simulink model "gm_sampleModel1444_3_sub"  (R2023a)
settings: Solver=VariableStepAuto  StartTime=0.0  StopTime=10.0  RelTol=1e-3
libraries: simulink x2, hdlsllib x1
settings Model: Creator=user1  LastModifiedBy=user1
settings OptimizationCC: BlockReduction=off  ConditionallyExecuteInputs=off
settings DebuggingCC: InheritedTsInSrcMsg=none

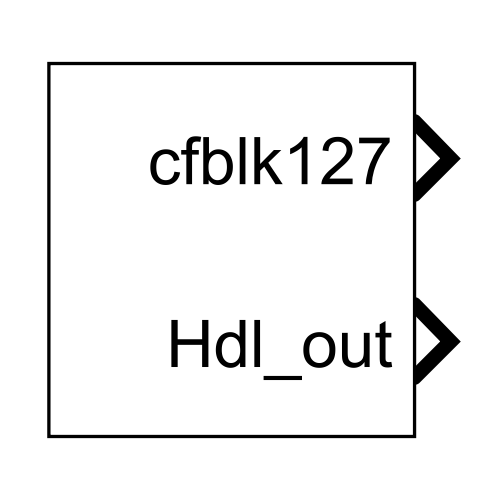
[thumbnail: Simulink's stored preview of the top-level diagram]
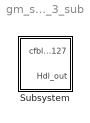
== system gm_sampleModel1444_3_sub ==
  Subsystem : Subsystem

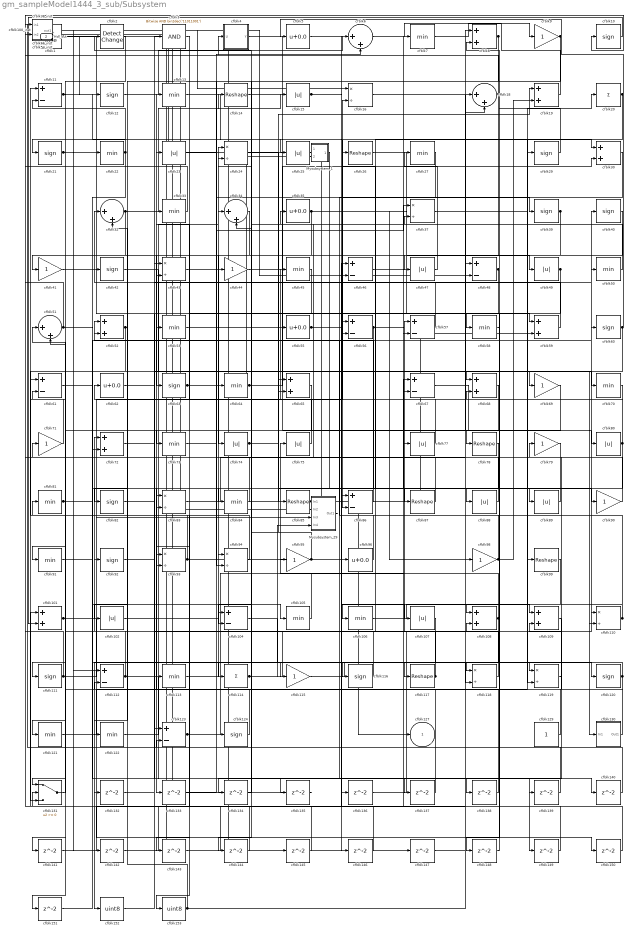
== system gm_sampleModel1444_3_sub/Subsystem ==
  Mysubsystem_1 : Subsystem
  Mysubsystem_29 : Subsystem
  cfblk1 : hdlsllib/Logic and Bit Operations/Bit Slice  lidx=7  ridx=0
  cfblk{10,12,21,29,39..40,42,60,63,82,92,111,116,120,124} (15 alike) : Signum
  cfblk100_inst : Subsystem
  cfblk{8,19,30,52,59,65,68,72,101,108..109} (11 alike) : Sum  OutDataTypeStr=uint8
  cfblk{15,23,25,47,49,74..75,77,80,88..89,102,107} (13 alike) : Abs  OutDataTypeStr=uint8  SaturateOnIntegerOverflow=off
  cfblk{11,46,48,56..57,61,67,86,104,112,123} (11 alike) : Sum  Inputs=+-  OutDataTypeStr=uint8
  cfblk{7,13,22,27,33,45,50,53,58,64,70,73,81,84,91,105..106,113,121..122} (20 alike) : MinMax  OutDataTypeStr=uint8
  cfblk{16,24,37,43,83,93..94,110,118..119} (10 alike) : Product  Inputs=*/  OutDataTypeStr=uint8  RndMeth=Zero  SaturateOnIntegerOverflow=on
  cfblk114 : Sum  Inputs=+  OutDataTypeStr=uint8
  cfblk{9,41,44,69,71,79,90,95,98,115} (10 alike) : Gain  OutDataTypeStr=uint8
  cfblk{14,26,78,85,87,99,117} (7 alike) : Reshape
  cfblk129 : Constant  OutDataTypeStr=uint8  SampleTime=-1
  cfblk130 : Subsystem
  cfblk131 : Switch  OutDataTypeStr=uint8  SaturateOnIntegerOverflow=off  InputSameDT=off
  cfblk{132..151} (20 alike) : Delay  SampleTime=1
  cfblk152 : DataTypeConversion  OutDataTypeStr=uint8  SaturateOnIntegerOverflow=off  RndMeth=Floor
  cfblk153 : DataTypeConversion  OutDataTypeStr=uint8  SaturateOnIntegerOverflow=off  RndMeth=Floor
  cfblk{6,18,32,34,51} (5 alike) : Sum  Inputs=|++  OutDataTypeStr=uint8
  cfblk2 : simulink/Logic and Bit Operations/Detect Change  vinit=0  OutDataTypeStr=uint8
      settings: LibrarySourceBlock=|
      | hdlsllib/Logic and Bit
      | Operations/Detect
      | Change
  cfblk20 : Sum  Inputs=+  OutDataTypeStr=uint8
  cfblk3 : simulink/Logic and Bit Operations/Bitwise Operator  logicop=AND  UseBitMask=on  BitMask=bin2dec('11011001')  BitMaskRealWorld=Stored Integer
      settings: LibrarySourceBlock=|
      | hdlsllib/Logic and Bit
      | Operations/Bitwise
      | Operator
  cfblk{5,35,55,62,96} (5 alike) : Bias  Bias=0.0  SaturateOnIntegerOverflow=off
  cfblk38_inst : Subsystem
  cfblk4 : Subsystem  mask(Detect Rise Nonnegative){vinit=double(0), InputProcessing=Elements as channels (sample based), OutDataTypeStr=uint8}
      mask prompts: vinit "Simulink:masks:InitialCondition_MP"; InputProcessing "Simulink:masks:InputProcessing_MP"; OutDataTypeStr "Simulink:masks:OutputDataType_MP"
      mask help: Simulink:masks:DetectRiseNonnegative_MD
      mask init:
      | InputProcessing = 'Elements as channels (sample based)';
      | OutDataTypeStr = 'uint8';
      | vinit = double(0);
      mask TypeOptions InputProcessing: Simulink:masks:ColumnsAsChannelsFrameBased | Simulink:masks:ElementsAsChannelsSampleBased
      mask TypeOptions OutDataTypeStr: Simulink:masks:uint8 | Simulink:masks:boolean
      mask Display: fprintf('U >= 0\n&  NOT\nU/z >= 0')
  cfblk54_inst : Subsystem
  cfblk66_inst : Subsystem
  cfblk127 : Outport  OutDataTypeStr=uint8  SampleTime=1  VectorParamsAs1DForOutWhenUnconnected=off
  Hdl_out : Outport  Port=2  OutDataTypeStr=uint8  SampleTime=1
  wires:
  Mysubsystem_1/1(Out1) -> cfblk133/1
  Mysubsystem_29/1(Out1) -> Mysubsystem_1/1(In1)
  cfblk1/1 -> cfblk86/2, cfblk12/1
  cfblk10/1 -> cfblk101/2
  cfblk100_inst/1(out1) -> cfblk48/2, Mysubsystem_29/2(In2)
  cfblk101/1 -> cfblk150/1, Mysubsystem_29/3(In3), cfblk105/1
  cfblk102/1 -> cfblk24/1
  cfblk104/1 -> cfblk119/1
  cfblk105/1 -> cfblk75/1
  cfblk106/1 -> cfblk109/1
  cfblk107/1 -> cfblk152/1
  cfblk108/1 -> cfblk95/1, cfblk132/1
  cfblk109/1 -> cfblk134/1
  cfblk11/1 -> cfblk30/1, cfblk151/1
  cfblk110/1 -> cfblk62/1, cfblk108/1
  cfblk111/1 -> cfblk10/1, cfblk16/2
  cfblk112/1 -> cfblk72/1, cfblk149/1
  cfblk113/1 -> cfblk94/1
  cfblk114/1 -> cfblk40/1, Mysubsystem_29/4(In4)
  cfblk115/1 -> cfblk120/1
  cfblk116/1 -> cfblk61/2
  cfblk117/1 -> cfblk92/1, cfblk57/1
  cfblk118/1 -> cfblk26/1
  cfblk119/1 -> cfblk79/1
  cfblk12/1 -> cfblk6/1
  cfblk120/1 -> cfblk116/1, cfblk112/2
  cfblk121/1 -> cfblk29/1
  cfblk122/1 -> cfblk34/1
  cfblk123/1 -> cfblk77/1, cfblk124/1
  cfblk124/1 -> cfblk13/1
  cfblk129/1 -> cfblk52/1
  cfblk13/1 -> cfblk96/1
  cfblk130/1(Out1) -> cfblk109/2
  cfblk131/1 -> cfblk81/1
  cfblk132/1 -> cfblk110/1
  cfblk133/1 -> cfblk6/2
  cfblk134/1 -> cfblk34/2
  cfblk135/1 -> cfblk1/1
  cfblk136/1 -> cfblk108/2
  cfblk137/1 -> cfblk93/2
  cfblk138/1 -> cfblk51/1
  cfblk139/1 -> cfblk100_inst/1(in1)
  cfblk14/1 -> cfblk146/1
  cfblk140/1 -> cfblk24/2
  cfblk141/1 -> cfblk67/1
  cfblk142/1 -> cfblk48/1
  cfblk143/1 -> cfblk46/1
  cfblk144/1 -> cfblk123/2
  cfblk145/1 -> cfblk66_inst/1(in1)
  cfblk146/1 -> cfblk101/1
  cfblk147/1 -> cfblk18/1
  cfblk148/1 -> cfblk8/2
  cfblk149/1 -> cfblk83/2
  cfblk15/1 -> cfblk59/1, cfblk69/1
  cfblk150/1 -> cfblk131/2
  cfblk151/1 -> cfblk56/2
  cfblk152/1 -> cfblk3/1
  cfblk153/1 -> cfblk52/2, cfblk18/2
  cfblk16/1 -> cfblk80/1
  cfblk18/1 -> cfblk131/1, cfblk4/1(U)
  cfblk19/1 -> cfblk7/1
  cfblk2/1 -> cfblk141/1
  cfblk20/1 -> cfblk86/1, cfblk119/2
  cfblk21/1 -> cfblk25/1, cfblk123/1
  cfblk22/1 -> cfblk72/2, cfblk21/1, cfblk11/2
  cfblk23/1 -> cfblk39/1
  cfblk24/1 -> cfblk56/1
  cfblk25/1 -> cfblk38_inst/2(in2)
  cfblk26/1 -> cfblk58/1
  cfblk27/1 -> cfblk46/2
  cfblk29/1 -> cfblk54_inst/1(in1)
  cfblk3/1 -> cfblk153/1
  cfblk30/1 -> cfblk115/1
  cfblk32/1 -> cfblk14/1, cfblk41/1
  cfblk33/1 -> cfblk100_inst/2(in2)
  cfblk34/1 -> cfblk63/1
  cfblk35/1 -> cfblk82/1, cfblk49/1, cfblk98/1
  cfblk37/1 -> cfblk20/1
  cfblk38_inst/1(out1) -> cfblk16/1, cfblk145/1, cfblk142/1
  cfblk39/1 -> cfblk47/1, cfblk37/2
  cfblk4/1(Y) -> cfblk99/1
  cfblk40/1 -> cfblk74/1
  cfblk41/1 -> cfblk85/1
  cfblk42/1 -> cfblk130/1(In1)
  cfblk43/1 -> cfblk64/1
  cfblk44/1 -> cfblk68/1
  cfblk45/1 -> cfblk143/1
  cfblk46/1 -> cfblk89/1
  cfblk47/1 -> cfblk27/1
  cfblk48/1 -> cfblk57/2, cfblk73/1
  cfblk49/1 -> cfblk104/2, cfblk148/1
  cfblk5/1 -> cfblk107/1
  cfblk50/1 -> cfblk2/1
  cfblk51/1 -> cfblk66_inst/2(in2), cfblk137/1
  cfblk52/1 -> cfblk32/2, cfblk121/1
  cfblk53/1 -> cfblk136/1
  cfblk54_inst/1(out1) -> cfblk147/1
  cfblk55/1 -> cfblk117/1, cfblk140/1
  cfblk56/1 -> cfblk93/1, cfblk90/1
  cfblk57/1 -> cfblk32/1
  cfblk58/1 -> cfblk138/1
  cfblk59/1 -> cfblk23/1
  cfblk6/1 -> cfblk67/2
  cfblk60/1 -> cfblk5/1, cfblk131/3
  cfblk61/1 -> cfblk53/1
  cfblk62/1 -> cfblk70/1
  cfblk63/1 -> cfblk37/1, Mysubsystem_1/2(In2)
  cfblk64/1 -> cfblk78/1, cfblk30/2
  cfblk65/1 -> cfblk91/1
  cfblk66_inst/1(out1) -> cfblk112/1, Mysubsystem_29/1(In1), cfblk22/1
  cfblk67/1 -> cfblk110/2
  cfblk68/1 -> cfblk122/1
  cfblk69/1 -> cfblk111/1
  cfblk7/1 -> cfblk9/1
  cfblk70/1 -> cfblk68/2
  cfblk71/1 -> cfblk11/1
  cfblk72/1 -> cfblk118/1
  cfblk73/1 -> cfblk15/1
  cfblk74/1 -> cfblk87/1, cfblk19/1
  cfblk75/1 -> cfblk43/2
  cfblk77/1 -> cfblk33/1
  cfblk78/1 -> cfblk114/1
  cfblk79/1 -> cfblk135/1
  cfblk8/1 -> cfblk102/1, cfblk94/2
  cfblk80/1 -> cfblk144/1, cfblk45/1
  cfblk81/1 -> cfblk104/1, cfblk83/1
  cfblk82/1 -> cfblk139/1
  cfblk83/1 -> cfblk8/1
  cfblk84/1 -> cfblk54_inst/2(in2)
  cfblk85/1 -> cfblk59/2, cfblk127/1
  cfblk86/1 -> cfblk42/1
  cfblk87/1 -> cfblk35/1
  cfblk88/1 -> cfblk38_inst/1(in1)
  cfblk89/1 -> cfblk88/1
  cfblk9/1 -> cfblk113/1, cfblk84/1
  cfblk90/1 -> cfblk43/1
  cfblk91/1 -> cfblk118/2
  cfblk92/1 -> cfblk50/1
  cfblk93/1 -> cfblk51/2, cfblk71/1
  cfblk94/1 -> cfblk61/1
  cfblk95/1 -> cfblk65/2, cfblk60/1, cfblk44/1, Hdl_out/1
  cfblk96/1 -> cfblk65/1
  cfblk98/1 -> cfblk55/1, cfblk19/2
  cfblk99/1 -> cfblk106/1

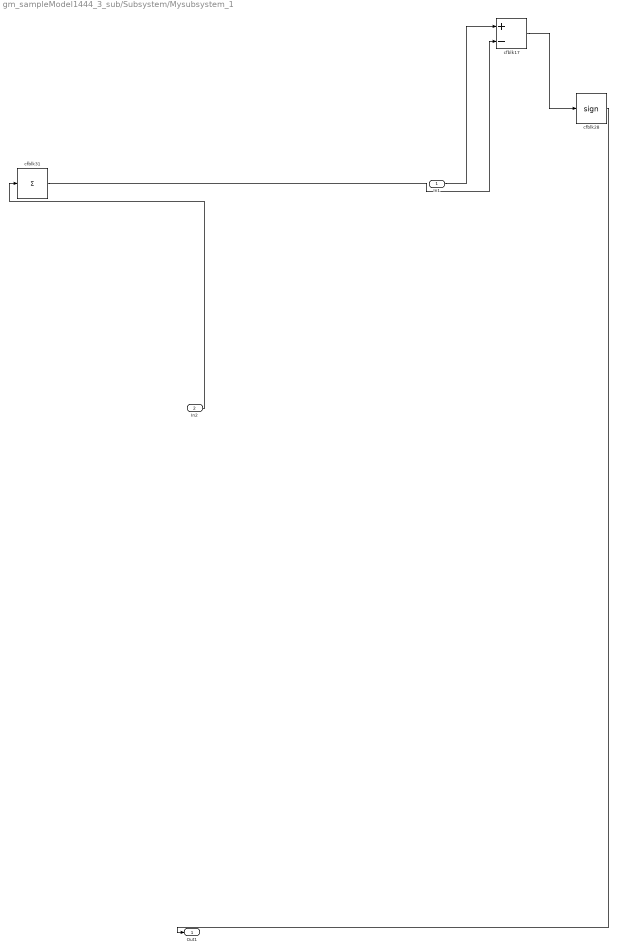
== system gm_sampleModel1444_3_sub/Subsystem/Mysubsystem_1 ==
  In1 : Inport  OutDataTypeStr=uint8  PortDimensions=1  SampleTime=1
  In2 : Inport  Port=2  OutDataTypeStr=uint8  PortDimensions=1  SampleTime=1
  cfblk17 : Sum  Inputs=+-
  cfblk28 : Signum
  cfblk31 : Sum  Inputs=+
  Out1 : Outport  SampleTime=1
  wires:
  In1/1 -> cfblk17/1
  In2/1 -> cfblk31/1
  cfblk17/1 -> cfblk28/1
  cfblk28/1 -> Out1/1
  cfblk31/1 -> cfblk17/2

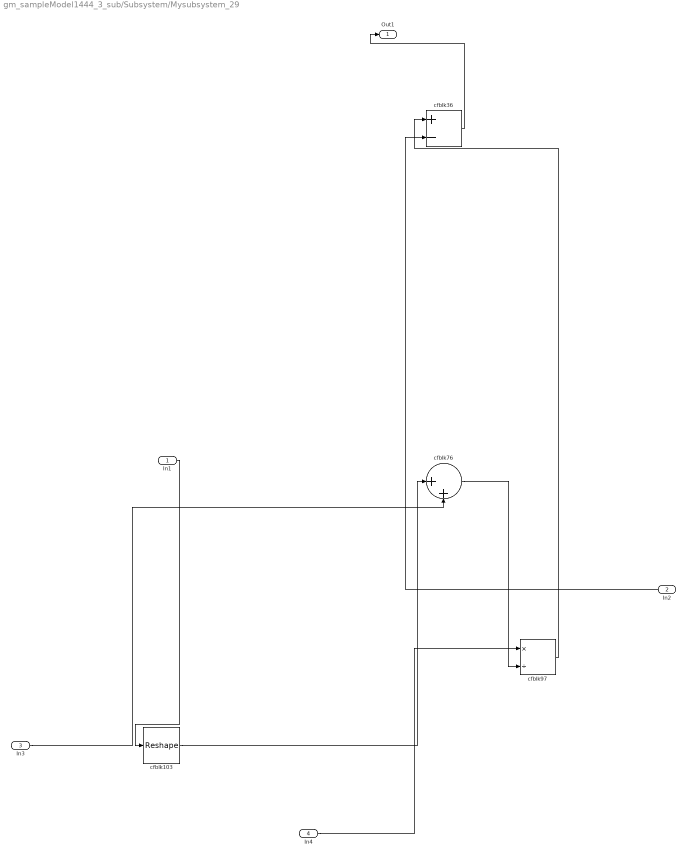
== system gm_sampleModel1444_3_sub/Subsystem/Mysubsystem_29 ==
  In1 : Inport  OutDataTypeStr=uint8  PortDimensions=1  SampleTime=1
  In2 : Inport  Port=2  OutDataTypeStr=uint8  PortDimensions=1  SampleTime=1
  In3 : Inport  Port=3  OutDataTypeStr=uint8  PortDimensions=1  SampleTime=1
  In4 : Inport  Port=4  OutDataTypeStr=uint8  PortDimensions=1  SampleTime=1
  cfblk103 : Reshape
  cfblk36 : Sum  Inputs=+-
  cfblk76 : Sum  Inputs=|++
  cfblk97 : Product  Inputs=*/  RndMeth=Zero  SaturateOnIntegerOverflow=on
  Out1 : Outport  SampleTime=1
  wires:
  In1/1 -> cfblk103/1
  In2/1 -> cfblk36/2
  In3/1 -> cfblk76/2
  In4/1 -> cfblk97/1
  cfblk103/1 -> cfblk76/1
  cfblk36/1 -> Out1/1
  cfblk76/1 -> cfblk97/2
  cfblk97/1 -> cfblk36/1

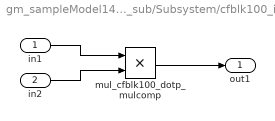
== system gm_sampleModel1444_3_sub/Subsystem/cfblk100_inst ==
  in1 : Inport  OutDataTypeStr=uint8  SampleTime=1
  in2 : Inport  Port=2  OutDataTypeStr=uint8  SampleTime=1
  mul_cfblk100_dotp_mulcomp : Product  Inputs=**  OutDataTypeStr=uint8  SampleTime=1
  out1 : Outport  OutDataTypeStr=uint8  SampleTime=1
  wires:
  in1/1 -> mul_cfblk100_dotp_mulcomp/1
  in2/1 -> mul_cfblk100_dotp_mulcomp/2
  mul_cfblk100_dotp_mulcomp/1 -> out1/1

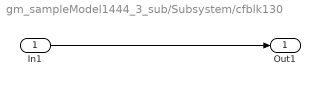
== system gm_sampleModel1444_3_sub/Subsystem/cfblk130 ==
  In1 : Inport  OutDataTypeStr=uint8  PortDimensions=1  SampleTime=1
  Out1 : Outport  SampleTime=1
  wires:
  In1/1 -> Out1/1

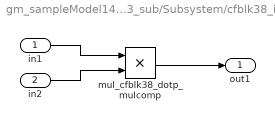
== system gm_sampleModel1444_3_sub/Subsystem/cfblk38_inst ==
  in1 : Inport  OutDataTypeStr=uint8  SampleTime=1
  in2 : Inport  Port=2  OutDataTypeStr=uint8  SampleTime=1
  mul_cfblk38_dotp_mulcomp : Product  Inputs=**  OutDataTypeStr=uint8  SampleTime=1
  out1 : Outport  OutDataTypeStr=uint8  SampleTime=1
  wires:
  in1/1 -> mul_cfblk38_dotp_mulcomp/1
  in2/1 -> mul_cfblk38_dotp_mulcomp/2
  mul_cfblk38_dotp_mulcomp/1 -> out1/1

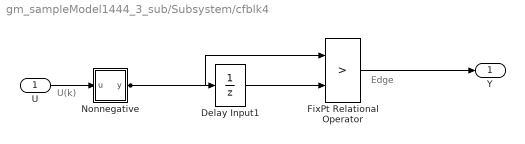
== system gm_sampleModel1444_3_sub/Subsystem/cfblk4 ==
  note: U(k)
  note: Edge
  U : Inport  OutDataTypeStr=uint8  SampleTime=1
  Delay Input1 : UnitDelay  Description=Store in Global RAM  DisableCoverage=on  InitialCondition=vinit  SampleTime=-1  HasFrameUpgradeWarning=on
  FixPt Relational Operator : RelationalOperator  Operator=>  OutDataTypeStr=fixdt(0, 8)  ZeroCross=off  InputSameDT=off
  Nonnegative : Subsystem  mask(Compare To Zero){relop=>=, OutDataTypeStr=boolean, ZeroCross=off}
      mask prompts: relop "Simulink:masks:Operator_MP"; OutDataTypeStr "Simulink:masks:OutputDataType_MP"; ZeroCross "Simulink:masks:EnableZerocrossingDetection_MP"
      mask help: Simulink:masks:CompareToZero_MD
      mask init:
      | OutDataTypeStr = 'boolean';
      | ZeroCross = 'off';
      | blkName = 'sampleModel1444_3_sub/Subsystem/cfblk4/Nonnegative';
      | relop = '>=';
      | setValue = 'boolean';
      mask TypeOptions relop: == | ~= | < | <= | >= | >
      mask TypeOptions OutDataTypeStr: Simulink:masks:uint8 | Simulink:masks:boolean
      mask Callback ZeroCross: sl('zeroCrossEnable', gcbh);
      mask Display: disp([relop,' 0'])
  Y : Outport  SampleTime=1
  wires:
  U/1 -> Nonnegative/1(u)
  Delay Input1/1 -> FixPt Relational Operator/2
  FixPt Relational Operator/1 -> Y/1
  Nonnegative/1(y) -> FixPt Relational Operator/1, Delay Input1/1

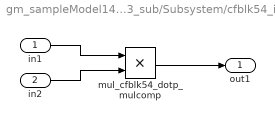
== system gm_sampleModel1444_3_sub/Subsystem/cfblk54_inst ==
  in1 : Inport  OutDataTypeStr=uint8  SampleTime=1
  in2 : Inport  Port=2  OutDataTypeStr=uint8  SampleTime=1
  mul_cfblk54_dotp_mulcomp : Product  Inputs=**  OutDataTypeStr=uint8  SampleTime=1
  out1 : Outport  OutDataTypeStr=uint8  SampleTime=1
  wires:
  in1/1 -> mul_cfblk54_dotp_mulcomp/1
  in2/1 -> mul_cfblk54_dotp_mulcomp/2
  mul_cfblk54_dotp_mulcomp/1 -> out1/1

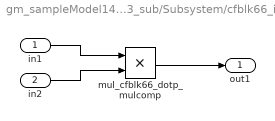
== system gm_sampleModel1444_3_sub/Subsystem/cfblk66_inst ==
  in1 : Inport  OutDataTypeStr=uint8  SampleTime=1
  in2 : Inport  Port=2  OutDataTypeStr=uint8  SampleTime=1
  mul_cfblk66_dotp_mulcomp : Product  Inputs=**  OutDataTypeStr=uint8  SampleTime=1
  out1 : Outport  OutDataTypeStr=uint8  SampleTime=1
  wires:
  in1/1 -> mul_cfblk66_dotp_mulcomp/1
  in2/1 -> mul_cfblk66_dotp_mulcomp/2
  mul_cfblk66_dotp_mulcomp/1 -> out1/1

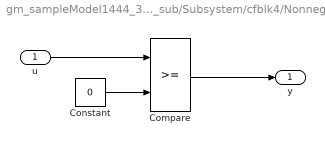
== system gm_sampleModel1444_3_sub/Subsystem/cfblk4/Nonnegative ==
  u : Inport  OutDataTypeStr=uint8  SampleTime=1
  Compare : RelationalOperator  OutDataTypeStr=boolean  ZeroCross=off
  Constant : Constant  DisableCoverage=on  Value=0  OutDataTypeStr=Inherit: Inherit via back propagation  SampleTime=-1  PreserveConstantTs=on
  y : Outport  SampleTime=1
  wires:
  u/1 -> Compare/1
  Compare/1 -> y/1
  Constant/1 -> Compare/2
